simulink model "quadrotor_model_with_payload"  (R2021a)
settings: Solver=FixedStepAuto  StartTime=0.0  StopTime=10.0  RelTol=1e-3
undefined symbols (not defined in the file): sim_freq, tau_w, v_gust
libraries: sharedtransform x2, shared6dof x1, simulink x1
settings Model: SimulationMode=accelerator  Creator=francois  LastModifiedBy=esl
settings SolverCC: ZeroCrossControl=DisableAll  AlgebraicLoopSolver=TrustRegion
settings DataIOCC: SaveOutput=off  SaveTime=off
settings DebuggingCC: SFMachineParentedDataDiag=warning
settings GRTTargetCC: CombineOutputUpdateFcns=off  MatFileLogging=off

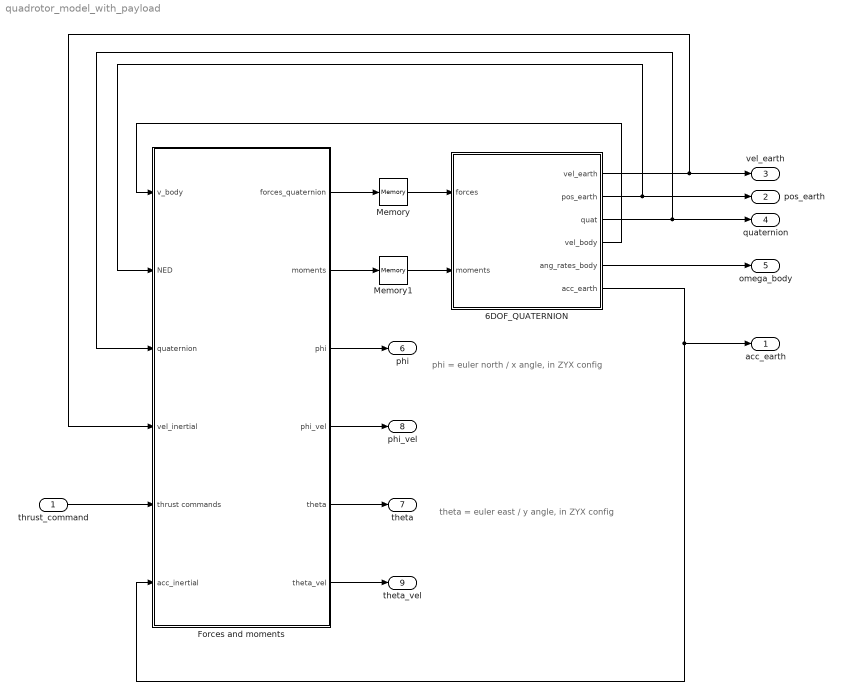
== system quadrotor_model_with_payload ==
  note: theta = euler east / y angle, in ZYX config
  note: phi = euler north / x angle, in ZYX config
  thrust_command : Inport  PortDimensions=4
  6DOF_QUATERNION : Subsystem
  "Forces and moments " : Subsystem
  Memory : Memory
  Memory1 : Memory
  acc_earth : Outport
  pos_earth : Outport  Port=2
  "vel_earth " : Outport  Port=3  PortDimensions=3
  quaternion : Outport  Port=4
  omega_body : Outport  Port=5
  phi : Outport  Port=6
  theta : Outport  Port=7
  phi_vel : Outport  Port=8
  theta_vel : Outport  Port=9
  wires:
  "Forces and moments "/1(forces_quaternion) -> Memory/1
  Memory1/1 -> 6DOF_QUATERNION/2(moments)
  6DOF_QUATERNION/5("ang_rates_body ") -> omega_body/1
  thrust_command/1 -> "Forces and moments "/5(thrust commands)
  6DOF_QUATERNION/1(vel_earth) -> "Forces and moments "/4(vel_inertial), "vel_earth "/1
  6DOF_QUATERNION/6("acc_earth ") -> "Forces and moments "/6(acc_inertial), acc_earth/1
  6DOF_QUATERNION/3(quat) -> "Forces and moments "/3(quaternion), quaternion/1
  Memory/1 -> 6DOF_QUATERNION/1(forces)
  6DOF_QUATERNION/4("vel_body ") -> "Forces and moments "/1(v_body)
  6DOF_QUATERNION/2(pos_earth) -> "Forces and moments "/2(NED), pos_earth/1
  "Forces and moments "/2(moments) -> Memory1/1
  "Forces and moments "/4(phi_vel) -> phi_vel/1
  "Forces and moments "/3(phi) -> phi/1
  "Forces and moments "/5(theta) -> theta/1
  "Forces and moments "/6(theta_vel) -> theta_vel/1

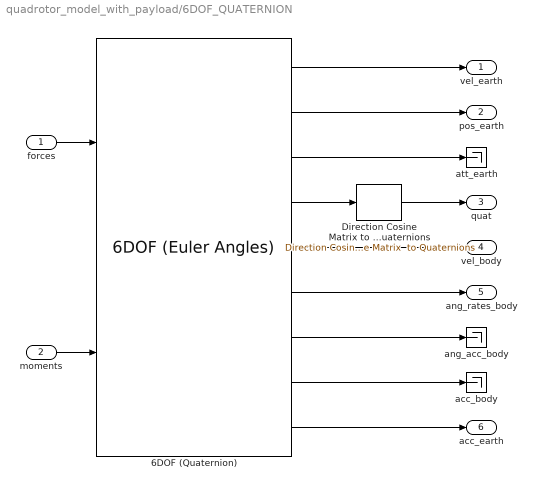
== system quadrotor_model_with_payload/6DOF_QUATERNION ==
  forces : Inport
  moments : Inport  Port=2
  6DOF (Quaternion) : shared6dof/6DOF (Euler Angles)  units=Metric (MKS)  mtype=Fixed  rep=Quaternion  xme_0=[0 0 0]  Vm_0=[0 0 0]  eul_0=[0 0 0]  pm_0=[0 0 0]  mass_0=mq  mass_e=0.5  mass_f=2.0  inertia=I  inertia_e=eye(3)  inertia_f=2*eye(3)  k_quat=2  vre_flag=on  abi_flag=on  aMode=0  xme_statename=''  Vm_statename=''  eul_statename=''  quat_statename=''  pm_statename=''  mass_statename=''
      settings: SourceProductBaseCode=AE,PW,DR,MT,UV,VE
  Direction Cosine Matrix to Quaternions : sharedtransform/Direction Cosine Matrix  to Quaternions  aMode=0  action=None  tolerance=eps(2)
      settings: SourceProductBaseCode=AE,PW,DR,MT,UV,VE
  acc_body : Terminator
  ang_acc_body : Terminator
  att_earth : Terminator
  vel_earth : Outport  PortDimensions=3
  pos_earth : Outport  Port=2
  quat : Outport  Port=3
  "vel_body " : Outport  Port=4
  "ang_rates_body " : Outport  Port=5
  "acc_earth " : Outport  Port=6
  wires:
  moments/1 -> 6DOF (Quaternion)/2
  6DOF (Quaternion)/7 -> ang_acc_body/1
  6DOF (Quaternion)/5 -> "vel_body "/1
  6DOF (Quaternion)/1 -> vel_earth/1
  forces/1 -> 6DOF (Quaternion)/1
  6DOF (Quaternion)/8 -> acc_body/1
  6DOF (Quaternion)/6 -> "ang_rates_body "/1
  6DOF (Quaternion)/3 -> att_earth/1
  6DOF (Quaternion)/2 -> pos_earth/1
  6DOF (Quaternion)/4 -> Direction Cosine Matrix to Quaternions/1
  Direction Cosine Matrix to Quaternions/1 -> quat/1
  6DOF (Quaternion)/9 -> "acc_earth "/1

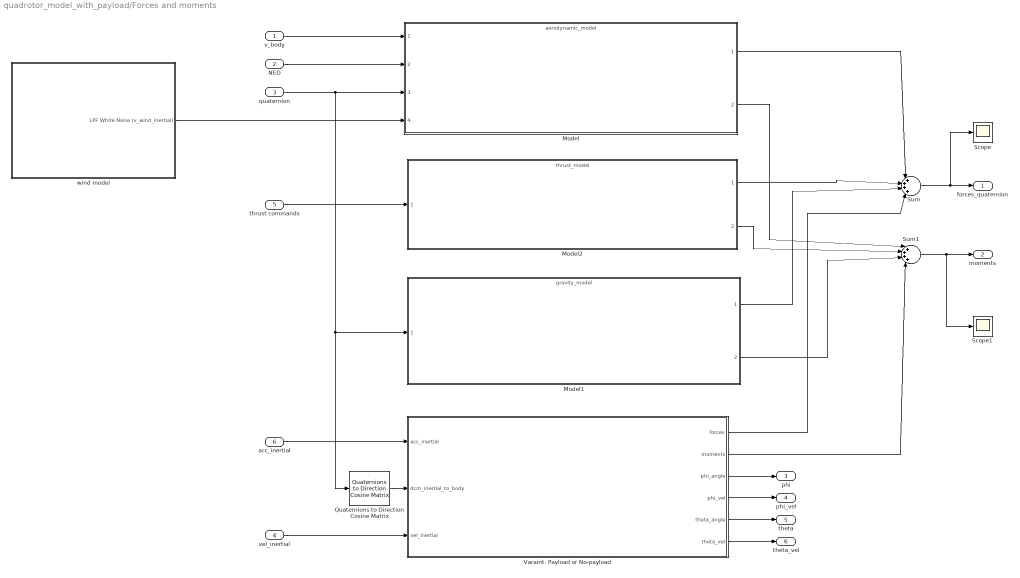
== system quadrotor_model_with_payload/Forces and moments  ==
  v_body : Inport  SampleTime=1/sim_freq
  NED : Inport  Port=2  SampleTime=1/sim_freq
  quaternion : Inport  Port=3  PortDimensions=4  SampleTime=1/sim_freq
  vel_inertial : Inport  Port=4  PortDimensions=3
  thrust commands : Inport  Port=5  PortDimensions=4  SampleTime=1/sim_freq
  acc_inertial : Inport  Port=6
  Model : ModelReference  ModelNameDialog=aerodynamic_model.slx  SimulationMode=Normal  ModelReferenceVersion=1.17
  Model1 : ModelReference  ModelNameDialog=gravity_model.slx  SimulationMode=Normal  ModelReferenceVersion=1.11
  Model2 : ModelReference  ModelNameDialog=thrust_model.slx  SimulationMode=Normal  ModelReferenceVersion=1.7
  Quaternions to Direction Cosine Matrix : sharedtransform/Quaternions to  Direction Cosine Matrix  aMode=aMode
      settings: SourceProductBaseCode=AE,PW,DR,MT,UV,VE
  Scope : Scope
  Scope1 : Scope
  Sum : Sum  Inputs=|++++|
  Sum1 : Sum  Inputs=|++++|
  Varaint: Payload or No-payload : Subsystem  Variant=on  AllowZeroVariantControls=on
  "wind model " : Subsystem
  forces_quaternion : Outport
  moments : Outport  Port=2
  phi : Outport  Port=3
  phi_vel : Outport  Port=4
  theta : Outport  Port=5
  theta_vel : Outport  Port=6
  wires:
  Sum1/1 -> Scope1/1, moments/1
  Sum/1 -> Scope/1, forces_quaternion/1
  thrust commands/1 -> Model2/1
  v_body/1 -> Model/1
  NED/1 -> Model/2
  quaternion/1 -> Model/3, Quaternions to Direction Cosine Matrix/1, Model1/1
  Model2/2 -> Sum1/2
  Model/2 -> Sum1/1
  Model2/1 -> Sum/2
  "wind model "/1(LPF White Noise (v_wind_inertial)) -> Model/4
  Model1/1 -> Sum/3
  Model1/2 -> Sum1/3
  acc_inertial/1 -> Varaint: Payload or No-payload/1(acc_inertial)
  Model/1 -> Sum/1
  vel_inertial/1 -> Varaint: Payload or No-payload/3(vel_inertial)
  Quaternions to Direction Cosine Matrix/1 -> Varaint: Payload or No-payload/2(dcm_inertial_to_body)
  Varaint: Payload or No-payload/3(phi_angle) -> phi/1
  Varaint: Payload or No-payload/4(phi_vel) -> phi_vel/1
  Varaint: Payload or No-payload/5(theta_angle) -> theta/1
  Varaint: Payload or No-payload/6(theta_vel) -> theta_vel/1
  Varaint: Payload or No-payload/2(moments) -> Sum1/4
  Varaint: Payload or No-payload/1(forces) -> Sum/4

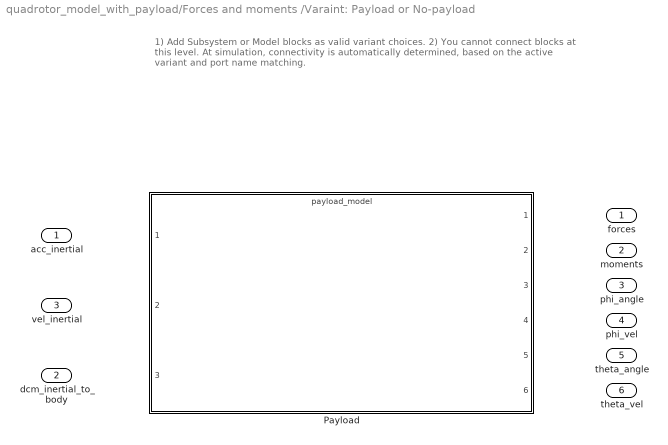
== system quadrotor_model_with_payload/Forces and moments /Varaint: Payload or No-payload ==
  note: 1) Add Subsystem or Model blocks as valid variant choices.
      | 2) You cannot connect blocks at this level. At simulation, connectivity is automatically
      | determined, based on the active variant and port name matching.
  acc_inertial : Inport  PortDimensions=3
  dcm_inertial_to_body : Inport  Port=2  PortDimensions=[3, 3]
  vel_inertial : Inport  Port=3  PortDimensions=3
  Payload : ModelReference  DisableCoverage=on  ModelNameDialog=payload_model.slx  VariantControl=payload_variant  ModelReferenceVersion=3.0
  forces : Outport  PortDimensions=3
  moments : Outport  Port=2  PortDimensions=3
  phi_angle : Outport  Port=3  PortDimensions=1
  phi_vel : Outport  Port=4  PortDimensions=1
  theta_angle : Outport  Port=5  PortDimensions=1
  theta_vel : Outport  Port=6  PortDimensions=1

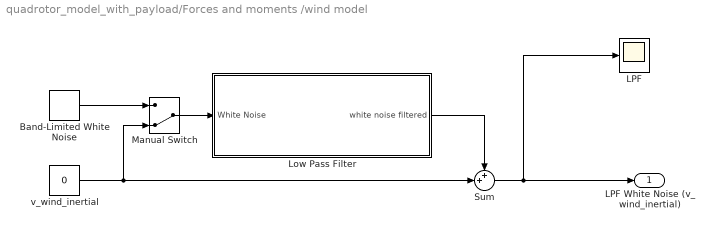
== system quadrotor_model_with_payload/Forces and moments /wind model  ==
  Band-Limited White Noise : simulink/Sources/Band-Limited White Noise  Cov=v_gust*ones(3,1)  Ts=1/sim_freq  seed=[23341]
  LPF : Scope
  "Low Pass Filter " : Subsystem
  Manual Switch : ManualSwitch  CurrentSetting=0
  Sum : Sum  Inputs=++|
  v_wind_inertial : Constant  Value=0
  LPF White Noise (v_wind_inertial) : Outport  PortDimensions=3
  wires:
  "Low Pass Filter "/1(white noise filtered) -> Sum/1
  v_wind_inertial/1 -> Manual Switch/2, Sum/2
  Sum/1 -> LPF/1, LPF White Noise (v_wind_inertial)/1
  Manual Switch/1 -> "Low Pass Filter "/1("White Noise ")
  Band-Limited White Noise/1 -> Manual Switch/1

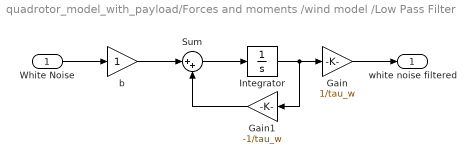
== system quadrotor_model_with_payload/Forces and moments /wind model /Low Pass Filter  ==
  "White Noise " : Inport
  Gain : Gain  Gain=1/tau_w
  Gain1 : Gain  Gain=-1/tau_w
  Integrator : Integrator
  Sum : Sum  Inputs=|++
  b : Gain
  white noise filtered : Outport
  wires:
  "White Noise "/1 -> b/1
  b/1 -> Sum/1
  Sum/1 -> Integrator/1
  Gain/1 -> white noise filtered/1
  Integrator/1 -> Gain/1, Gain1/1
  Gain1/1 -> Sum/2
